simulink model "multivariate_gaussian_sampling"  (R2021b)
settings: Solver=FixedStepDiscrete  StartTime=0.0  StopTime=100.0  RelTol=1e-3
libraries: wnnutils x2, wnnsinks x2, wnnsources x1
settings Model: Creator=20214358  LastModifiedBy=20214358

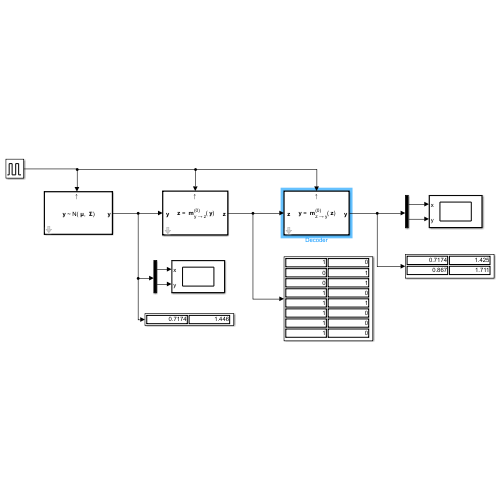
[thumbnail: Simulink's stored preview of the top-level diagram]
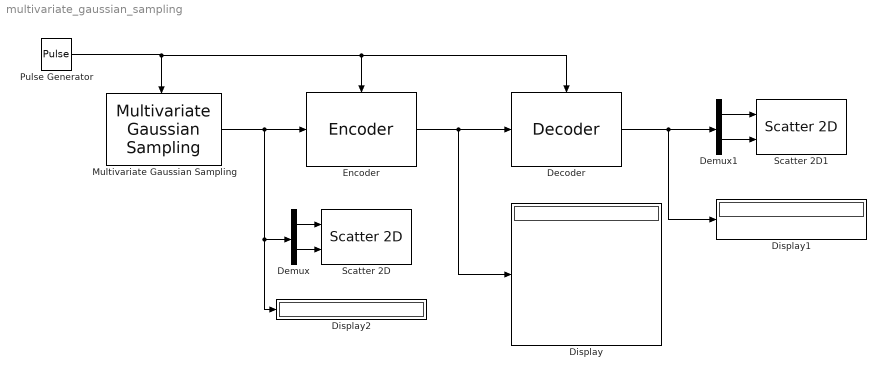
== system multivariate_gaussian_sampling ==
  Decoder : wnnutils/Decoder  encoder_id=0  output_dims=2
  Demux : Demux  Outputs=2
  Demux1 : Demux  Outputs=2
  Display : Display
  Display1 : Display
  Display2 : Display
  Encoder : wnnutils/Encoder  encoder_id=0  output_dims=16  learning_rate=0.001  min_splitting_volume=0.01  min_bounds="[-10  -10]"  max_bounds=[10 10]
  Multivariate Gaussian Sampling : wnnsources/Multivariate Gaussian Sampling  vecdAvg=[1 1]  matdCov=[2 1; 1 2]  nSeed=0
  Pulse Generator : DiscretePulseGenerator  PulseType=Time based  Period=1  PulseWidth=5
  Scatter 2D : wnnsinks/Scatter 2D  SystemSampleTime=-1  VariantActivationTime=update diagram  Latency=0  AutoFrameSizeCalculation=off
  Scatter 2D1 : wnnsinks/Scatter 2D  SystemSampleTime=-1  VariantActivationTime=update diagram  Latency=0  AutoFrameSizeCalculation=off
  wires:
  Pulse Generator/1 -> Decoder/Trigger, Encoder/Trigger, Multivariate Gaussian Sampling/Trigger
  Demux/1 -> Scatter 2D/1
  Demux/2 -> Scatter 2D/2
  Multivariate Gaussian Sampling/1 -> Display2/1, Demux/1, Encoder/1
  Demux1/2 -> Scatter 2D1/2
  Demux1/1 -> Scatter 2D1/1
  Encoder/1 -> Display/1, Decoder/1
  Decoder/1 -> Display1/1, Demux1/1
